simulink model "Zustandsregelung_mit_Vorsteuerung_linear"  (R2021b)
settings: Solver=FixedStepAuto  StartTime=0.0  StopTime=10  FixedStep=1/1e4  RelTol=1e-3
undefined symbols (not defined in the file): A, B, C, d, delta_y_ref_Vor, F, k_LMI_2, x_Ruhe
settings Model: Creator=basti  LastModifiedBy=basti

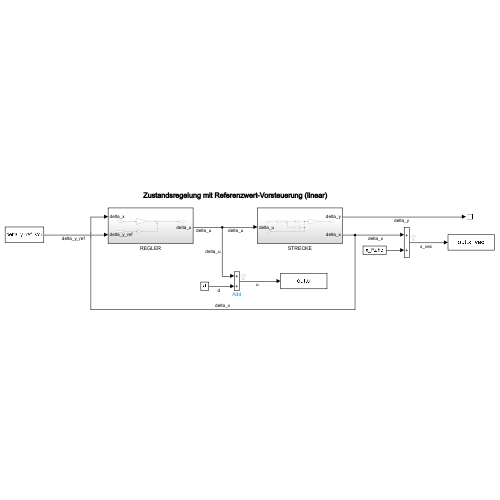
[thumbnail: Simulink's stored preview of the top-level diagram]
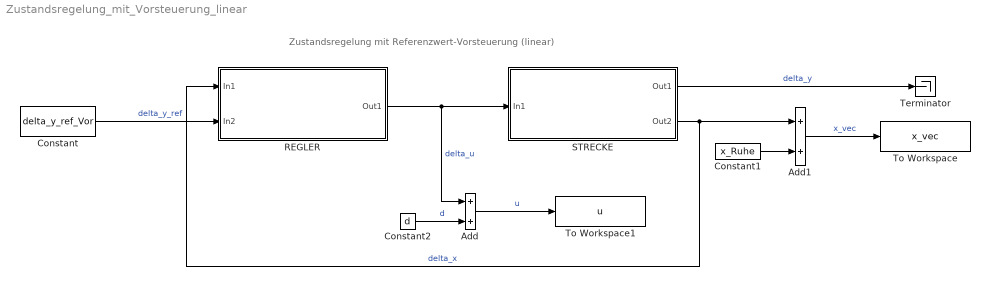
== system Zustandsregelung_mit_Vorsteuerung_linear ==
  note: Zustandsregelung mit Referenzwert-Vorsteuerung (linear)
  Add : Sum
  Add1 : Sum
  Constant : Constant  Value=delta_y_ref_Vor
  Constant1 : Constant  Value=x_Ruhe
  Constant2 : Constant  Value=d
  REGLER : Subsystem
  STRECKE : Subsystem
  Terminator : Terminator
  To Workspace : ToWorkspace  VariableName=x_vec  SaveFormat=Timeseries  SampleTime=-1
  To Workspace1 : ToWorkspace  VariableName=u  SaveFormat=Timeseries  SampleTime=-1
  wires:
  STRECKE/1(Out1) -> Terminator/1  "delta_y"
  Constant/1 -> REGLER/2(In2)  "delta_y_ref"
  Add1/1 -> To Workspace/1  "x_vec"
  Constant1/1 -> Add1/2
  STRECKE/2(Out2) -> Add1/1, REGLER/1(In1)  "delta_x"
  Constant2/1 -> Add/2  "d"
  REGLER/1(Out1) -> Add/1, STRECKE/1(In1)  "delta_u"
  Add/1 -> To Workspace1/1  "u"

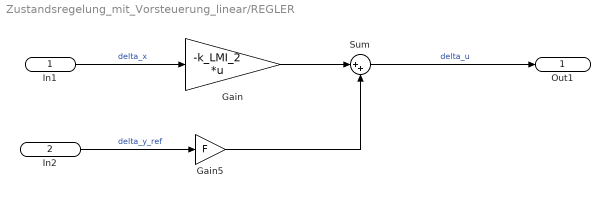
== system Zustandsregelung_mit_Vorsteuerung_linear/REGLER ==
  In1 : Inport
  In2 : Inport  Port=2
  Gain : Gain  Gain=-k_LMI_2  Multiplication=Matrix(K*u) (u vector)
  Gain5 : Gain  Gain=F
  Sum : Sum  Inputs=|++
  Out1 : Outport
  wires:
  Gain/1 -> Sum/1
  In1/1 -> Gain/1  "delta_x"
  Gain5/1 -> Sum/2
  In2/1 -> Gain5/1  "delta_y_ref"
  Sum/1 -> Out1/1  "delta_u"

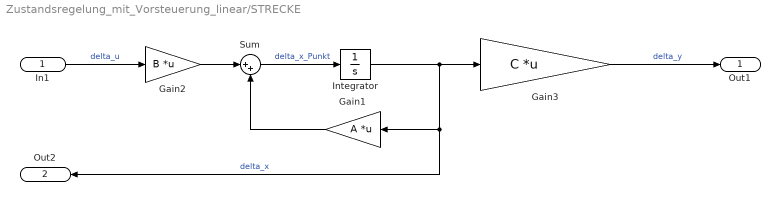
== system Zustandsregelung_mit_Vorsteuerung_linear/STRECKE ==
  In1 : Inport
  Gain1 : Gain  Gain=A  Multiplication=Matrix(K*u) (u vector)
  Gain2 : Gain  Gain=B  Multiplication=Matrix(K*u) (u vector)
  Gain3 : Gain  Gain=C  Multiplication=Matrix(K*u) (u vector)
  Integrator : Integrator
  Sum : Sum  Inputs=|++
  Out1 : Outport
  Out2 : Outport  Port=2
  wires:
  Gain1/1 -> Sum/2
  Gain3/1 -> Out1/1  "delta_y"
  Sum/1 -> Integrator/1  "delta_x_Punkt"
  Integrator/1 -> Out2/1, Gain1/1, Gain3/1  "delta_x"
  Gain2/1 -> Sum/1
  In1/1 -> Gain2/1  "delta_u"
